simulink subsystem "Memristor_NonVolatile_Subsystem"  (R2024b)
settings: Solver=VariableStepAuto  StartTime=0.0  StopTime=10.0  RelTol=1e-3
libraries: fl_lib x4, nesl_utility x3
settings Model: DefaultTestHarness=Memristor_NonVolatile_Subsystem_Harness1  Creator=georg  LastModifiedBy=georg

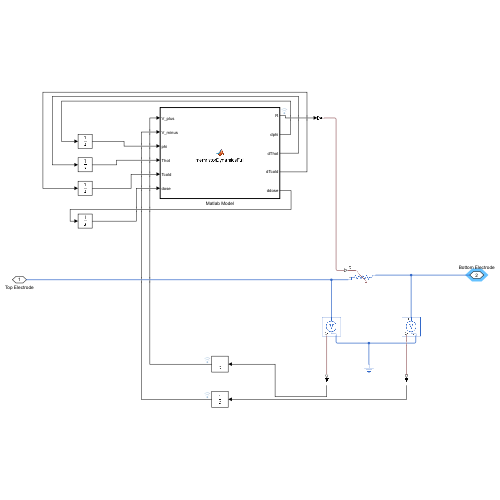
[thumbnail: Simulink's stored preview of the top-level diagram]
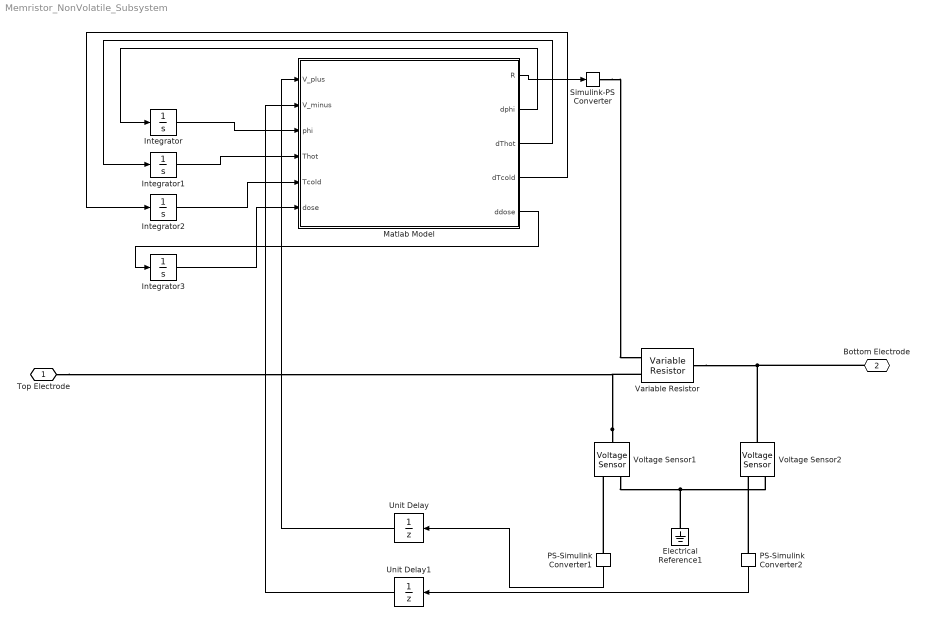
== system Memristor_NonVolatile_Subsystem ==
  Electrical Reference1 : fl_lib/Electrical/Electrical Elements/Electrical Reference
  Integrator : Integrator  InitialCondition=0.24e-09
  Integrator1 : Integrator  InitialCondition=300
  Integrator2 : Integrator  InitialCondition=300
  Integrator3 : Integrator
  Matlab Model : MATLAB Function  TreatAsAtomicUnit=on
  PS-Simulink Converter1 : nesl_utility/PS-Simulink Converter  PhysicalDomain=network_engine_domain  SubClassName=ps_output  LeftPortType=input  RightPortType=output  PseudoPeriodic=off  Frequencies=[]  VectorFormat=inherit  Unit=inherit  AffineConversion=off
  PS-Simulink Converter2 : nesl_utility/PS-Simulink Converter  PhysicalDomain=network_engine_domain  SubClassName=ps_output  LeftPortType=input  RightPortType=output  PseudoPeriodic=off  Frequencies=[]  VectorFormat=inherit  Unit=inherit  AffineConversion=off
  Simulink-PS Converter : nesl_utility/Simulink-PS Converter  PhysicalDomain=network_engine_domain  SubClassName=ps_input  LeftPortType=input  RightPortType=output  PseudoPeriodic=off  Frequencies=[]  NoiseDistribution=none  NoiseParameters=[]  Unit=1  AffineConversion=off  FilteringAndDerivatives=filter  SimscapeFilterOrder=1  InputFilterTimeConstant=0.00001  UdotUserProvided=0
  Unit Delay : UnitDelay  SampleTime=-1  HasFrameUpgradeWarning=on
  Unit Delay1 : UnitDelay  SampleTime=-1  HasFrameUpgradeWarning=on
  Variable Resistor : fl_lib/Electrical/Electrical Elements/Variable Resistor  Rmin=0 kOhm  thermalEnable=false  thermal_mass=1 J/K  i_specify=off  i_priority=None  i=0 A  i_nominal_specify=off  i_nominal_value=1  i_nominal_unit=A  v_specify=off  v_priority=None  v=0 V  v_nominal_specify=off  v_nominal_value=1  v_nominal_unit=V  T_specify=off  T_priority=None  T=300 K  T_nominal_specify=off  T_nominal_value=1  T_nominal_unit=K
  Voltage Sensor1 : fl_lib/Electrical/Electrical Sensors/Voltage Sensor
  Voltage Sensor2 : fl_lib/Electrical/Electrical Sensors/Voltage Sensor
  Top Electrode : PMIOPort  Side=Left
  Bottom Electrode : PMIOPort  Port=2  Side=Right
  wires:
  PS-Simulink Converter2/1 -> Unit Delay1/1
  Matlab Model/2(dphi) -> Integrator/1
  Integrator1/1 -> Matlab Model/4(Thot)
  Matlab Model/3(dThot) -> Integrator1/1
  Matlab Model/4(dTcold) -> Integrator2/1
  Integrator/1 -> Matlab Model/3(phi)
  Unit Delay1/1 -> Matlab Model/2(V_minus)
  Matlab Model/1(R) -> Simulink-PS Converter/1
  Matlab Model/5(ddose) -> Integrator3/1
  Integrator2/1 -> Matlab Model/5(Tcold)
  Integrator3/1 -> Matlab Model/6(dose)
  Unit Delay/1 -> Matlab Model/1(V_plus)
  PS-Simulink Converter1/1 -> Unit Delay/1
  connections:
  Electrical Reference1/LConn1 -- Voltage Sensor1/RConn2 -- Voltage Sensor2/RConn2
  Voltage Sensor2/LConn1 -- Bottom Electrode/RConn1 -- Variable Resistor/RConn1
  Voltage Sensor1/LConn1 -- Top Electrode/RConn1 -- Variable Resistor/LConn2
  PS-Simulink Converter1/LConn1 -- Voltage Sensor1/RConn1
  PS-Simulink Converter2/LConn1 -- Voltage Sensor2/RConn1
  Simulink-PS Converter/RConn1 -- Variable Resistor/LConn1

== matlab function Memristor_NonVolatile_Subsystem/Matlab Model ==
  data: V_plus input; V_minus input; R output; phi input; Thot input; Tcold input; dphi output; dThot output; dTcold output; dose input; ddose output
function [R, dphi, dThot, dTcold, ddose] = memristorDynamicsFull(V_plus, V_minus, phi, Thot, Tcold, dose)
% Inputs: voltage terminals, state variables (phi, Thot, Tcold, dose)
% Outputs: resistance R, and derivatives of each state variable

% === Voltage ===
V = V_plus - V_minus;

% === Model Constants ===
q     = 1.602176634e-19;
kb    = 1.38064852e-23;
rT    = 20e-9;
rB    = 4e-9;
L     = 20e-9;
g     = 1e-9;
phi_max = 12e-9;
phi_min = 0.01e-9;
Tamb  = 300;
Tau_th = 2.3e-9;
m     = 2000e-9;
rbulkm = 3e-13;
rbulkox = 1000;
gamma  = 20e-9;
el    = 28e-9;
p     = 0.5;
AP    = 1.5;
BP    = 1e-4;
CP    = 1.2e-24;
Edrift = 1.15 * q;
Ediff  = 2.5 * q;
alphaP = 1.0;
Aexp  = 0.5;
Es    = 0.8 * q;
phi_sat = 2e-9;
phi_B = 0.65 * q;
A_star = 1.2e6;
n_schottky = 1.5;
lambda_plasticity = 100;
gamma_dose = 1;
T_trigger = 400;
T_slope = 20;
Vmax = 2;
Km = 1e-15;
healing_rate = 1;

% === Utility functions ===
st_f = @(y, y0) 1 / (1 + exp(-y / y0));
soft_barrier = @(y, width) 1 / (1 + (y / width)^2);

% === Resistance ===
S = Es / (kb * Thot^2);
E = V / g;
rx1 = rT - ((rT - phi/2) / (L/2)) * ((L/2) - g);
rx2 = rB - ((rB - phi/2) / (L/2)) * ((L/2) - g);
rcf = rbulkm * (1 + (3/4)*(el/phi)*(1 - p));
rox = rbulkox / (1 + gamma*abs(E));

Roff = (rcf*(L-g)/(2*pi*rT*rx1)) + ...
       (rcf*(L-g)/(2*pi*rB*rx2)) + ...
       (rox * g / (pi * rx1 * rx2));
Ron = (rcf * L / (2*pi*rT*phi/2)) + ...
      (rcf * L / (2*pi*rB*phi/2));
R = st_f(phi - phi_max, 1e-9) * Ron + ...
    st_f(phi_min - phi, 1e-9) * Roff;

% === Currents ===
phi_limit = 0.2e-9;
Area_eff = pi * (min(phi, phi_limit)/2)^2;
J0 = A_star * Thot^2 * exp(-phi_B / (kb * Thot));
J_schottky = J0 * (exp(q*V / (n_schottky*kb*Thot)) - 1);
I_schottky = J_schottky * Area_eff;
I_cf = V / R;
I_total = I_cf + I_schottky;

% === Thermal dynamics ===
kthcold = m * (2 * rT);
kthhot = m * phi;
dTcold = (abs(V * I_total) / kthcold + Tamb / Tau_th - Tcold / Tau_th);
dThot  = (abs(V * I_total) / kthhot + Tamb / Tau_th - Thot / Tau_th);
deltaT = Thot - Tcold;
T = Thot;

% === State derivatives ===
drift = AP * exp(-Aexp * (Edrift - alphaP * q * V) / (kb * T)) * st_f(V, 0.2) * soft_barrier(phi - phi_max, 1e-2);
diff = BP * (1/phi) * exp(-Ediff / (kb*T)) * (1 + gamma_dose*dose) * exp(-phi / phi_sat);
thermal = CP * S * (1/phi) * deltaT / (L/2) * (1 + lambda_plasticity * dose) * exp(phi_min/phi);
thermal = thermal * (1 + (0.5 + 0.5*tanh((deltaT - T_trigger) / T_slope)));
neg_drift = AP * exp(-Aexp * (Edrift - alphaP*q*abs(V)) / (kb*T)) * ...
            st_f(-V, 0.2) * st_f(phi - phi_max, 1e-9);

dphi = st_f(phi_max - phi, 1e-10) * (drift + diff - thermal) - ...
       st_f(phi - phi_min, 1e-10) * (diff + neg_drift + thermal);

% === Dose (plasticity) ===
absorbed_energy = abs(V * I_total);
temperature_factor = max((T - Tamb), 0) / Tamb;
dose_rate = (Vmax * absorbed_energy * temperature_factor) / ...
            (Km + absorbed_energy * temperature_factor);
healing_effect = exp(-(Tcold - Tamb) / 10);
ddose = dose_rate - healing_rate * healing_effect * dose;

end






% function [R, dphi, dThot, dTcold] = memristorDynamics(V_plus, V_minus, phi, Thot, Tcold)
% function [R, dphi, dThot, dTcold] = memristorDynamics(V_plus, V_minus, phi, Thot, Tcold)
% %MEMRISTORDYNAMICS Memristor model from voltage and internal states.
% %   Inputs:
% %     V      - Voltage across memristor (V)
% %     phi    - Filament diameter (m)
% %     Thot   - Hot-side temperature (K)
% %     Tcold  - Cold-side temperature (K)
% %   Outputs:
% %     R      - Memristance (Ohms)
% %     dphi   - Time derivative of phi (m/s)
% %     dThot  - Time derivative of Thot (K/s)
% %     dTcold - Time derivative of Tcold (K/s)
% V = V_plus - V_minus;
% % -------------------------
% % Constants
% % -------------------------
% rT = 10E-9; 
% rB = 4E-9; 
% L = 20E-9; 
% g = 10E-9;
% Tamb = 300; 
% kth = 20; 
% m = 2000E-9;
% q = 1.602176634E-19; 
% kb = 1.38064852E-23;
% Edrift = 1.25 * q; 
% Ediff = 1.5 * q; 
% Es = 1 * q;
% alphaP = 5.8; 
% BP = 1E-5; 
% CP = 0.9E-25; 
% AP = 0.5;
% rbulkm = 3E-9; 
% rbulkox = 15; 
% gamma = 1E-9; 
% p = 0.5; 
% el = 28E-9; 
% fiat = 0.25E-9;
% Tau_th = 2.3e-10;
% 
% % -------------------------
% % Geometry-based resistance
% % -------------------------
% rx1 = rT - ((rT - (phi / 2)) / (L / 2)) * ((L / 2) - g);
% rx2 = rB - ((rB - (phi / 2)) / (L / 2)) * ((L / 2) - g);
% rcf = rbulkm * (1 + (3/4) * (el / phi) * (1 - p));
% 
% E = V / g;
% rox = rbulkox / (1 + gamma * abs(E));
% 
% Roff = ((rcf * (L - g) / 2) / (pi * rT * rx1) + ...
%         (rcf * (L - g) / 2) / (pi * rB * rx2) + ...
%         (rox * g) / (pi * rx1 * rx2));
% Ron = ((rcf * L / 2) / (pi * rT * phi / 2) + ...
%        (rcf * L / 2) / (pi * rB * phi / 2));
% 
% s_on = 1 / (1 + exp(-(phi - fiat) / 1e-15));
% s_off = 1 - s_on;
% R = s_on * Ron + s_off * Roff;
% 
% % -------------------------
% % Temperature dynamics
% % -------------------------
% power = abs(V)^2 / R;
% kthcold = m * (2 * rT);
% kthhot = m * phi;
% 
% dTcold = (power / kthcold + Tamb / Tau_th - Tcold / Tau_th);
% dThot = (power / kthhot + Tamb / Tau_th - Thot / Tau_th);
% 
% T = Thot;
% S = Es / (kb * T^2);
% 
% % -------------------------
% % Filament evolution
% % -------------------------
% drift = AP * exp(-(Edrift - alphaP * q * V) / (kb * T));
% diff = BP * (1 / phi) * exp(-Ediff / (kb * T));
% thermal = CP * S * (1 / phi) * (Thot - Tcold) / (L / 2);
% 
% f1 = 1 / (1 + exp(-(2e-9 - phi) / 1e-12));
% f2 = 1 / (1 + exp(-(phi - 0.01e-9) / 1e-12));
% 
% dphi = (f1 * (drift + diff) - f2 * thermal);
% end
